simulink model "sysgenImageDoubleBuffer"  (Simulink 7.7)
settings: Solver=VariableStepDiscrete  StartTime=0.0  StopTime=((c_rx_rows_2*c_rx_cols_2)*2+(320*10))+5000  RelTol=1e-3
PreLoadFcn:
  | sysgenImageDoubleBuffer_PreLoadFcn
StartFcn:
  | tic;
undefined symbols (not defined in the file or in its folder): c_rx_cols_1, c_rx_cols_2, c_rx_rows_1, c_rx_rows_2, dpost_1, dpost_2
libraries: xbsIndex_r4 x160, dspbuff3 x6, dspsigattribs x6, dspmtrx3 x6, vipsrcs x2, simulink x2, xbsCopyrightNotice_r4 x1
(part 2 of 3)

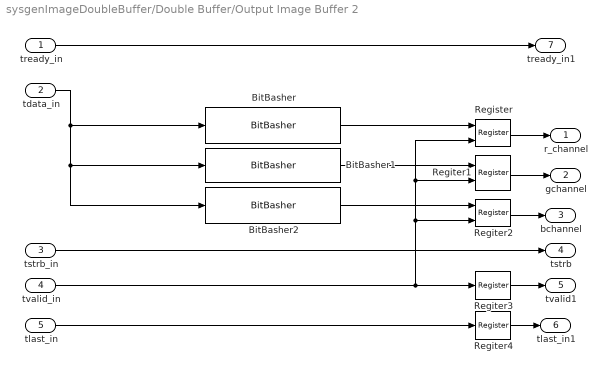
== system sysgenImageDoubleBuffer/Double Buffer/Output Image Buffer 2 ==
  tready_in : Inport
  tdata_in : Inport  Port=2
  tstrb_in : Inport  Port=3
  tvalid_in : Inport  Port=4
  tlast_in : Inport  Port=5
  BitBasher : xbsIndex_r4/BitBasher  bitexpr=|  display_expr=off  sr_1=1  arith_type1=Unsigned  bin_pt1=0  sr_2=2  arith_type2=Unsigned  bin_pt2=0  sr_3=3  arith_type3=Unsigned  bin_pt3=0  sr_4=4  arith_type4=Unsigned  bin_pt4=0  dbl_ovrd=off  block_type=bitbasher
      | <!DOCTYPE HTML PUBLIC "-//W3C//DTD HTML 4.0//EN" "http://www.w3.org/TR/REC-html40/strict.dtd">
      | <html><head><meta name="qrichtext" content="1" /><style type="text/css">
      | p, li { white-space: pre-wrap; }
      | </style></head><body style=" font-family:'MS Shell Dlg 2'; font-size:7.8pt; font-weight:400; font-style:normal;">
      | <p style=" margin-top:12px; margin-bottom:12px; margin-left:0px; margin-right:0px; -qt-block-indent:0; text-indent:0px;"><span style=" font-family:'MS Shell Dlg'; font-size:8pt;">r_channel={mem[23:16]}</span></p></body></html>
      settings: block_version=12.3
  BitBasher1 : xbsIndex_r4/BitBasher  bitexpr=|  display_expr=off  sr_1=1  arith_type1=Unsigned  bin_pt1=0  sr_2=2  arith_type2=Unsigned  bin_pt2=0  sr_3=3  arith_type3=Unsigned  bin_pt3=0  sr_4=4  arith_type4=Unsigned  bin_pt4=0  dbl_ovrd=off  block_type=bitbasher
      | <!DOCTYPE HTML PUBLIC "-//W3C//DTD HTML 4.0//EN" "http://www.w3.org/TR/REC-html40/strict.dtd">
      | <html><head><meta name="qrichtext" content="1" /><style type="text/css">
      | p, li { white-space: pre-wrap; }
      | </style></head><body style=" font-family:'MS Shell Dlg 2'; font-size:7.8pt; font-weight:400; font-style:normal;">
      | <p style=" margin-top:12px; margin-bottom:12px; margin-left:0px; margin-right:0px; -qt-block-indent:0; text-indent:0px;"><span style=" font-family:'MS Shell Dlg'; font-size:8pt;">g_channel={mem[15:8]}</span></p></body></html>
      settings: block_version=12.3
  BitBasher2 : xbsIndex_r4/BitBasher  bitexpr=|  display_expr=off  sr_1=1  arith_type1=Unsigned  bin_pt1=0  sr_2=2  arith_type2=Unsigned  bin_pt2=0  sr_3=3  arith_type3=Unsigned  bin_pt3=0  sr_4=4  arith_type4=Unsigned  bin_pt4=0  dbl_ovrd=off  block_type=bitbasher
      | <!DOCTYPE HTML PUBLIC "-//W3C//DTD HTML 4.0//EN" "http://www.w3.org/TR/REC-html40/strict.dtd">
      | <html><head><meta name="qrichtext" content="1" /><style type="text/css">
      | p, li { white-space: pre-wrap; }
      | </style></head><body style=" font-family:'MS Shell Dlg 2'; font-size:7.8pt; font-weight:400; font-style:normal;">
      | <p style=" margin-top:12px; margin-bottom:12px; margin-left:0px; margin-right:0px; -qt-block-indent:0; text-indent:0px;"><span style=" font-family:'MS Shell Dlg'; font-size:8pt;">b_channel={mem[7:0]}</span></p></body></html>
      settings: block_version=12.3
  Register : xbsIndex_r4/Register  init=0  rst=off  en=on  dbl_ovrd=off  block_type=register
      settings: block_version=12.3
  Regiter1 : xbsIndex_r4/Register  init=0  rst=off  en=on  dbl_ovrd=off  block_type=register
      settings: block_version=12.3
  Regiter2 : xbsIndex_r4/Register  init=0  rst=off  en=on  dbl_ovrd=off  block_type=register
      settings: block_version=12.3
  Regiter3 : xbsIndex_r4/Register  init=0  rst=off  en=off  dbl_ovrd=off  block_type=register
      settings: block_version=12.3
  Regiter4 : xbsIndex_r4/Register  init=0  rst=off  en=off  dbl_ovrd=off  block_type=register
      settings: block_version=12.3
  r_channel : Outport
  gchannel : Outport  Port=2
  bchannel : Outport  Port=3
  tstrb : Outport  Port=4
  tvalid1 : Outport  Port=5
  tlast_in1 : Outport  Port=6
  tready_in1 : Outport  Port=7
  wires:
  tready_in/1 -> tready_in1/1
  tvalid_in/1 -> Regiter2/2, Regiter1/2, Register/2, Regiter3/1
  tdata_in/1 -> BitBasher/1, BitBasher1/1, BitBasher2/1
  BitBasher/1 -> Register/1
  BitBasher1/1 -> Regiter1/1
  BitBasher2/1 -> Regiter2/1
  Register/1 -> r_channel/1
  Regiter1/1 -> gchannel/1
  Regiter2/1 -> bchannel/1
  Regiter3/1 -> tvalid1/1
  tlast_in/1 -> Regiter4/1
  Regiter4/1 -> tlast_in1/1
  tstrb_in/1 -> tstrb/1

== system sysgenImageDoubleBuffer/Image_Source_1/Image_source_1 ==
  valid_push : Inport
  valid_pop : Inport  Port=2
  B_Queue : dspbuff3/Queue  depth=9999999  trigger=Non-zero sample  overflow=Dynamic reallocation  pes=Warning  eso=off  fso=off  nso=off  clr=off  clrOutport=off  adf=on
  G_Queue : dspbuff3/Queue  depth=9999999  trigger=Non-zero sample  overflow=Dynamic reallocation  pes=Warning  eso=off  fso=off  nso=off  clr=off  clrOutport=off  adf=on
  R_Queue : dspbuff3/Queue  depth=9999999  trigger=Non-zero sample  overflow=Dynamic reallocation  pes=Warning  eso=off  fso=off  nso=off  clr=off  clrOutport=off  adf=on
  Subsystem1 : Subsystem
  r_channel : Outport
  g_channel : Outport  Port=2
  b_channel : Outport  Port=3
  wires:
  Subsystem1/1(r_channel) -> R_Queue/1
  Subsystem1/2(g_channel) -> G_Queue/1
  Subsystem1/3(b_channel) -> B_Queue/1
  R_Queue/1 -> r_channel/1
  G_Queue/1 -> g_channel/1
  B_Queue/1 -> b_channel/1
  valid_push/1 -> R_Queue/2, G_Queue/2, B_Queue/2
  valid_pop/1 -> R_Queue/3, G_Queue/3, B_Queue/3

== system sysgenImageDoubleBuffer/Image_Source_1/Subsystem1 ==
  ready : Inport
  aresetn : Inport  Port=2
  Data Type Conversion : DataTypeConversion
  Logical Operator : Logic  IconShape=distinctive  AllPortsSameDT=off
  Logical Operator1 : Logic  Operator=NOT  AllPortsSameDT=off  OutDataTypeStr=boolean
  Logical Operator2 : Logic  IconShape=distinctive  AllPortsSameDT=off
  image frame valid : Subsystem
  valid_push : Outport
  valid_pop : Outport  Port=2
  transmit_image_1 : Outport  Port=3
  wires:
  ready/1 -> Logical Operator/1
  Logical Operator/1 -> Data Type Conversion/1
  Logical Operator2/1 -> Logical Operator/2, Logical Operator1/1
  Logical Operator1/1 -> transmit_image_1/1
  Data Type Conversion/1 -> valid_pop/1
  image frame valid/1(Out1) -> Logical Operator2/1, valid_push/1
  aresetn/1 -> Logical Operator2/2

== system sysgenImageDoubleBuffer/image_Source_2/Subsystem ==
  ready : Inport
  aresetn : Inport  Port=2
  Data Type Conversion : DataTypeConversion
  Logical Operator : Logic  IconShape=distinctive  AllPortsSameDT=off
  Logical Operator1 : Logic  Operator=NOT  AllPortsSameDT=off  OutDataTypeStr=boolean
  Logical Operator2 : Logic  IconShape=distinctive  AllPortsSameDT=off
  image frame valid : Subsystem
  valid_push : Outport
  valid_pop : Outport  Port=2
  transmit_image_2 : Outport  Port=3
  wires:
  ready/1 -> Logical Operator/1
  Logical Operator/1 -> Data Type Conversion/1
  Logical Operator2/1 -> Logical Operator/2, Logical Operator1/1
  Logical Operator1/1 -> transmit_image_2/1
  Data Type Conversion/1 -> valid_pop/1
  aresetn/1 -> Logical Operator2/2
  image frame valid/1(Out1) -> Logical Operator2/1, valid_push/1

== system sysgenImageDoubleBuffer/image_Source_2/image_source_2 ==
  valid_push : Inport
  valid_pop : Inport  Port=2
  B_Queue : dspbuff3/Queue  depth=9999999  trigger=Non-zero sample  overflow=Dynamic reallocation  pes=Warning  eso=off  fso=off  nso=off  clr=off  clrOutport=off  adf=on
  G_Queue : dspbuff3/Queue  depth=9999999  trigger=Non-zero sample  overflow=Dynamic reallocation  pes=Warning  eso=off  fso=off  nso=off  clr=off  clrOutport=off  adf=on
  R_Queue : dspbuff3/Queue  depth=9999999  trigger=Non-zero sample  overflow=Dynamic reallocation  pes=Warning  eso=off  fso=off  nso=off  clr=off  clrOutport=off  adf=on
  Subsystem3 : Subsystem
  r_channel : Outport
  g_channel : Outport  Port=2
  b_channel : Outport  Port=3
  wires:
  Subsystem3/1(r_channel) -> R_Queue/1
  Subsystem3/2(g_channel) -> G_Queue/1
  Subsystem3/3(b_channel) -> B_Queue/1
  R_Queue/1 -> r_channel/1
  valid_push/1 -> R_Queue/2, G_Queue/2, B_Queue/2
  valid_pop/1 -> R_Queue/3, G_Queue/3, B_Queue/3
  G_Queue/1 -> g_channel/1
  B_Queue/1 -> b_channel/1

== system sysgenImageDoubleBuffer/Double Buffer/Double Buffer/Block Descriptor Generator ==
  note: This subsystem is composed of two units :
      | xldScatterGatherEngineLineTransfer : This unit interfaces with the Master AXI Read Channel
      | hence it provides a Slave AXI Read Channel. It provides data transfer commands in the form
      | of Block Descriptors to enable line transfers of the input image.
      | xldScatterGatherEngineBlockTransfer : This unit interfaces with the Master AXI Read Channel
      | hence it provides a Slave AXI Read Channel. It provides data transfer commands in the form
      | of Block Descriptors to enable Tile transfers of the input image.
  axi_read_channel_in : Inport
  image1_switch_to_transmit : Inport  Port=2
  Bus Creator3 : BusCreator  Inputs=5
  Constant : xbsIndex_r4/Constant  const=tx_rows_1  gui_display_data_type=Fixed-point  arith_type=Unsigned  n_bits=16  bin_pt=0  preci_type=Single  exp_width=8  frac_width=24  explicit_period=off  period=1  equ=P=C  opselect=C  inp2=PCIN>>17  opr=+  inp1=P  carry=CIN  dbl_ovrd=off  block_type=constant
      settings: block_version=12.3
  Constant2 : xbsIndex_r4/Constant  const=tx_cols_1  gui_display_data_type=Fixed-point  arith_type=Unsigned  n_bits=16  bin_pt=0  preci_type=Single  exp_width=8  frac_width=24  explicit_period=off  period=1  equ=P=C  opselect=C  inp2=PCIN>>17  opr=+  inp1=P  carry=CIN  dbl_ovrd=off  block_type=constant
      settings: block_version=12.3
  Demux2 : Demux  Outputs=8  BusSelectionMode=on
  Expression1 : xbsIndex_r4/Expression  expression=~a  align_bp=on  en=off  latency=0  precision=Full  arith_type=Unsigned  n_bits=16  bin_pt=0  dbl_ovrd=off  block_type=expr
      settings: block_version=13.4
  Receiver Block Descriptor Generator : xbsIndex_r4/MCode  mfname=xldScatterGatherEngineLineTransfer_1  explicit_period=on  period=1  inputsTable={'boundInpExpr'=>['','','','','','','','','rx_rows_1','rx_cols_1'],'inputs'=>['araddr','arlen','arsize','arburst','arprot','arcache','arvalid','rready','rx_rows','rx_cols']}  outputsTable={'outputs'=>['arready','rvalid','rlast','rdata','rresp'],'suppressOut'=>['off','off','off','off','off']}  dbl_ovrd=off  enable_stdout=off  enable_debug=off  suppress_output=on  defparams={'rx_rows',rx_rows_1,'rx_cols',rx_cols_1}  hide_port_list={}  block_type=mcode
      settings: block_version=12.3
  Subsystem : Subsystem
  Subsystem1 : Subsystem
  Subsystem4 : Subsystem
  Transmitter Block Descriptor Generator1 : xbsIndex_r4/MCode  mfname=xldScatterGatherEngineBlockTransfer_1  explicit_period=on  period=1  inputsTable={'boundInpExpr'=>['','','','','','','','','tx_rows_1','tx_cols_1'],'inputs'=>['araddr','arlen','arsize','arburst','arprot','arcache','arvalid','rready','tx_rows','tx_cols']}  outputsTable={'outputs'=>['arready','rvalid','rlast','rdata','rresp'],'suppressOut'=>['off','off','off','off','off']}  dbl_ovrd=off  enable_stdout=off  enable_debug=off  suppress_output=on  defparams={'tx_rows',tx_rows_1,'tx_cols',tx_cols_1}  hide_port_list={}  block_type=mcode
      settings: block_version=12.3
  axi_read_channel_out : Outport
  tx_rows_1 : Outport  Port=2
  tx_cols_1 : Outport  Port=3
  wires:
  image1_switch_to_transmit/1 -> Subsystem/1(gate), Subsystem1/1(gate), Expression1/1
  Subsystem/1(araddr) -> Receiver Block Descriptor Generator/1
  Subsystem/2(arlen) -> Receiver Block Descriptor Generator/2
  Subsystem/3(arsize) -> Receiver Block Descriptor Generator/3
  Subsystem/4(arburst) -> Receiver Block Descriptor Generator/4
  Subsystem/5(arprot) -> Receiver Block Descriptor Generator/5
  Subsystem/6(arcache) -> Receiver Block Descriptor Generator/6
  Subsystem/7(arvalid) -> Receiver Block Descriptor Generator/7
  Subsystem/8(rready) -> Receiver Block Descriptor Generator/8
  Demux2/1 -> Subsystem/2(araddr_in), Subsystem4/2(araddr_in)
  Demux2/2 -> Subsystem/3(arlen_in), Subsystem4/3(arlen_in)
  Demux2/3 -> Subsystem/4(arsize_in), Subsystem4/4(arsize_in)
  Demux2/4 -> Subsystem/5(arburst_in), Subsystem4/5(arburst_in)
  Demux2/5 -> Subsystem/6(arprot_in), Subsystem4/6(arprot_in)
  Demux2/6 -> Subsystem/7(arcache_in), Subsystem4/7(arcache_in)
  Demux2/7 -> Subsystem/8(arvalid_in), Subsystem4/8(arvalid_in)
  Demux2/8 -> Subsystem/9(rready_in), Subsystem4/9(rready_in)
  Subsystem4/1(araddr) -> Transmitter Block Descriptor Generator1/1
  Subsystem4/2(arlen) -> Transmitter Block Descriptor Generator1/2
  Subsystem4/3(arsize) -> Transmitter Block Descriptor Generator1/3
  Subsystem4/4(arburst) -> Transmitter Block Descriptor Generator1/4
  Subsystem4/5(arprot) -> Transmitter Block Descriptor Generator1/5
  Subsystem4/6(arcache) -> Transmitter Block Descriptor Generator1/6
  Subsystem4/7(arvalid) -> Transmitter Block Descriptor Generator1/7
  Subsystem4/8(rready) -> Transmitter Block Descriptor Generator1/8
  Receiver Block Descriptor Generator/1 -> Subsystem1/2(arready_1)
  Transmitter Block Descriptor Generator1/1 -> Subsystem1/7(arready_2)
  Receiver Block Descriptor Generator/2 -> Subsystem1/3(rvalid_1)
  Transmitter Block Descriptor Generator1/2 -> Subsystem1/8(rvalid_2)
  Receiver Block Descriptor Generator/3 -> Subsystem1/4(rlast_1)
  Transmitter Block Descriptor Generator1/3 -> Subsystem1/9(rlast_2)
  Receiver Block Descriptor Generator/4 -> Subsystem1/5(rdata_1)
  Transmitter Block Descriptor Generator1/4 -> Subsystem1/10(rdata_2)
  Transmitter Block Descriptor Generator1/5 -> Subsystem1/11(rresp_2)
  Receiver Block Descriptor Generator/5 -> Subsystem1/6(rresp_1)
  Subsystem1/1(arready) -> Bus Creator3/1
  Subsystem1/2(rvalid) -> Bus Creator3/2
  Subsystem1/3(rlast) -> Bus Creator3/3
  Subsystem1/4(rdata) -> Bus Creator3/4
  Subsystem1/5(rresp) -> Bus Creator3/5
  Bus Creator3/1 -> axi_read_channel_out/1
  axi_read_channel_in/1 -> Demux2/1
  Expression1/1 -> Subsystem4/1(gate)
  Constant/1 -> tx_rows_1/1
  Constant2/1 -> tx_cols_1/1

== system sysgenImageDoubleBuffer/Double Buffer/Double Buffer/Block Descriptor Generator1 ==
  note: This subsystem is composed of two units :
      | xldScatterGatherEngineLineTransfer : This unit interfaces with the Master AXI Read Channel
      | hence it provides a Slave AXI Read Channel. It provides data transfer commands in the form
      | of Block Descriptors to enable line transfers of the input image.
      | xldScatterGatherEngineBlockTransfer : This unit interfaces with the Master AXI Read Channel
      | hence it provides a Slave AXI Read Channel. It provides data transfer commands in the form
      | of Block Descriptors to enable Tile transfers of the input image.
  axi_read_channel_in : Inport
  image2_switch_to_transmit : Inport  Port=2
  Bus Creator3 : BusCreator  Inputs=5
  Constant3 : xbsIndex_r4/Constant  const=tx_rows_2  gui_display_data_type=Fixed-point  arith_type=Unsigned  n_bits=16  bin_pt=0  preci_type=Single  exp_width=8  frac_width=24  explicit_period=off  period=1  equ=P=C  opselect=C  inp2=PCIN>>17  opr=+  inp1=P  carry=CIN  dbl_ovrd=off  block_type=constant
      settings: block_version=12.3
  Constant4 : xbsIndex_r4/Constant  const=tx_cols_2  gui_display_data_type=Fixed-point  arith_type=Unsigned  n_bits=16  bin_pt=0  preci_type=Single  exp_width=8  frac_width=24  explicit_period=off  period=1  equ=P=C  opselect=C  inp2=PCIN>>17  opr=+  inp1=P  carry=CIN  dbl_ovrd=off  block_type=constant
      settings: block_version=12.3
  Constant7 : xbsIndex_r4/Constant  const=rx_rows_2  gui_display_data_type=Fixed-point  arith_type=Unsigned  n_bits=16  bin_pt=0  preci_type=Single  exp_width=8  frac_width=24  explicit_period=off  period=1  equ=P=C  opselect=C  inp2=PCIN>>17  opr=+  inp1=P  carry=CIN  dbl_ovrd=off  block_type=constant
      settings: block_version=12.3
  Constant8 : xbsIndex_r4/Constant  const=rx_cols_2  gui_display_data_type=Fixed-point  arith_type=Unsigned  n_bits=16  bin_pt=0  preci_type=Single  exp_width=8  frac_width=24  explicit_period=off  period=1  equ=P=C  opselect=C  inp2=PCIN>>17  opr=+  inp1=P  carry=CIN  dbl_ovrd=off  block_type=constant
      settings: block_version=12.3
  Demux2 : Demux  Outputs=8  BusSelectionMode=on
  Expression1 : xbsIndex_r4/Expression  expression=~a  align_bp=on  en=off  latency=0  precision=Full  arith_type=Unsigned  n_bits=16  bin_pt=0  dbl_ovrd=off  block_type=expr
      settings: block_version=13.4
  Receiver Block Descriptor Generator : xbsIndex_r4/MCode  mfname=xldScatterGatherEngineLineTransfer_2  explicit_period=on  period=1  inputsTable={'boundInpExpr'=>['','','','','','','','','rx_rows_2','rx_cols_2'],'inputs'=>['araddr','arlen','arsize','arburst','arprot','arcache','arvalid','rready','rx_rows','rx_cols']}  outputsTable={'outputs'=>['arready','rvalid','rlast','rdata','rresp'],'suppressOut'=>['off','off','off','off','off']}  dbl_ovrd=off  enable_stdout=off  enable_debug=off  suppress_output=on  defparams={'rx_rows',rx_rows_2,'rx_cols',rx_cols_2}  hide_port_list={}  block_type=mcode
      settings: block_version=12.3
  Subsystem : Subsystem
  Subsystem1 : Subsystem
  Subsystem4 : Subsystem
  Transmitter Block Descriptor Generator1 : xbsIndex_r4/MCode  mfname=xldScatterGatherEngineBlockTransfer_2  explicit_period=on  period=1  inputsTable={'boundInpExpr'=>['','','','','','','','','tx_rows_2','tx_cols_2','rx_rows_2','rx_cols_2'],'inputs'=>['araddr','arlen','arsize','arburst','arprot','arcache','arvalid','rready','tx_rows','tx_cols','rx_rows','rx_cols']}  outputsTable={'outputs'=>['arready','rvalid','rlast','rdata','rresp'],'suppressOut'=>['off','off','off','off','off']}  dbl_ovrd=off  enable_stdout=off  enable_debug=off  suppress_output=on  defparams={'tx_rows',tx_rows_2,'tx_cols',tx_cols_2,'rx_rows',rx_rows_2,'rx_cols',rx_cols_2}  hide_port_list={}  block_type=mcode
      settings: block_version=12.3
  axi_read_channel_out : Outport
  tx_rows_2 : Outport  Port=2
  tx_cols_2 : Outport  Port=3
  rx_rows_2 : Outport  Port=4
  rx_cols_2 : Outport  Port=5
  wires:
  image2_switch_to_transmit/1 -> Subsystem1/1(gate), Subsystem/1(gate), Expression1/1
  Subsystem/1(araddr) -> Receiver Block Descriptor Generator/1
  Subsystem/2(arlen) -> Receiver Block Descriptor Generator/2
  Subsystem/3(arsize) -> Receiver Block Descriptor Generator/3
  Subsystem/4(arburst) -> Receiver Block Descriptor Generator/4
  Subsystem/5(arprot) -> Receiver Block Descriptor Generator/5
  Subsystem/6(arcache) -> Receiver Block Descriptor Generator/6
  Subsystem/7(arvalid) -> Receiver Block Descriptor Generator/7
  Subsystem/8(rready) -> Receiver Block Descriptor Generator/8
  Demux2/1 -> Subsystem/2(araddr_in), Subsystem4/2(araddr_in)
  Demux2/2 -> Subsystem/3(arlen_in), Subsystem4/3(arlen_in)
  Demux2/3 -> Subsystem/4(arsize_in), Subsystem4/4(arsize_in)
  Demux2/4 -> Subsystem/5(arburst_in), Subsystem4/5(arburst_in)
  Demux2/5 -> Subsystem/6(arprot_in), Subsystem4/6(arprot_in)
  Demux2/6 -> Subsystem/7(arcache_in), Subsystem4/7(arcache_in)
  Demux2/7 -> Subsystem/8(arvalid_in), Subsystem4/8(arvalid_in)
  Demux2/8 -> Subsystem/9(rready_in), Subsystem4/9(rready_in)
  Subsystem4/1(araddr) -> Transmitter Block Descriptor Generator1/1
  Subsystem4/2(arlen) -> Transmitter Block Descriptor Generator1/2
  Subsystem4/3(arsize) -> Transmitter Block Descriptor Generator1/3
  Subsystem4/4(arburst) -> Transmitter Block Descriptor Generator1/4
  Subsystem4/5(arprot) -> Transmitter Block Descriptor Generator1/5
  Subsystem4/6(arcache) -> Transmitter Block Descriptor Generator1/6
  Subsystem4/7(arvalid) -> Transmitter Block Descriptor Generator1/7
  Subsystem4/8(rready) -> Transmitter Block Descriptor Generator1/8
  Receiver Block Descriptor Generator/1 -> Subsystem1/2(arready_1)
  Transmitter Block Descriptor Generator1/1 -> Subsystem1/7(arready_2)
  Receiver Block Descriptor Generator/2 -> Subsystem1/3(rvalid_1)
  Transmitter Block Descriptor Generator1/2 -> Subsystem1/8(rvalid_2)
  Receiver Block Descriptor Generator/3 -> Subsystem1/4(rlast_1)
  Transmitter Block Descriptor Generator1/3 -> Subsystem1/9(rlast_2)
  Receiver Block Descriptor Generator/4 -> Subsystem1/5(rdata_1)
  Transmitter Block Descriptor Generator1/4 -> Subsystem1/10(rdata_2)
  Transmitter Block Descriptor Generator1/5 -> Subsystem1/11(rresp_2)
  Receiver Block Descriptor Generator/5 -> Subsystem1/6(rresp_1)
  Subsystem1/1(arready) -> Bus Creator3/1
  Subsystem1/2(rvalid) -> Bus Creator3/2
  Subsystem1/3(rlast) -> Bus Creator3/3
  Subsystem1/4(rdata) -> Bus Creator3/4
  Subsystem1/5(rresp) -> Bus Creator3/5
  Bus Creator3/1 -> axi_read_channel_out/1
  axi_read_channel_in/1 -> Demux2/1
  Expression1/1 -> Subsystem4/1(gate)
  Constant3/1 -> tx_rows_2/1
  Constant4/1 -> tx_cols_2/1
  Constant7/1 -> rx_rows_2/1
  Constant8/1 -> rx_cols_2/1

== system sysgenImageDoubleBuffer/Double Buffer/Double Buffer/Control Instructions Generator ==
  note: This block configures the VDMA as Reciever and
      | then as transmitter of image data. It interfaces with
      |  the Slave AXI Lite control interface of the VDMA,
      | hence it provides an Master AXI Lite Interface
  axi_lite_channel_in : Inport
  image1_switch_to_transmit : Inport  Port=2
  aresetn : Inport  Port=3
  Bus Creator1 : BusCreator  Inputs=8
  Control Command Generator : xbsIndex_r4/MCode  mfname=xlWriteControlRegister_db  explicit_period=on  period=1  inputsTable={'boundInpExpr'=>['','','','','','','','','',''],'inputs'=>['awready','wready','bresp','bvalid','arready','rvalid','rdata','rresp','switch_to_transmit','aresetn']}  outputsTable={'outputs'=>['awvalid','awaddr','wvalid','wdata','bready','arvalid','araddr','rready'],'suppressOut'=>['off','off','off','off','off','off','off','off']}  dbl_ovrd=off  enable_stdout=off  enable_debug=off  suppress_output=on  defparams={}  hide_port_list={}  block_type=mcode
      settings: block_version=12.3
  Demux : Demux  Outputs=8  BusSelectionMode=on
  axi_lite_channel_out : Outport
  wires:
  Demux/1 -> Control Command Generator/1
  Demux/2 -> Control Command Generator/2
  Demux/3 -> Control Command Generator/3
  Demux/4 -> Control Command Generator/4
  Demux/5 -> Control Command Generator/5
  Demux/6 -> Control Command Generator/6
  Demux/7 -> Control Command Generator/7
  Demux/8 -> Control Command Generator/8
  Control Command Generator/1 -> Bus Creator1/1
  Control Command Generator/2 -> Bus Creator1/2
  Control Command Generator/3 -> Bus Creator1/3
  Control Command Generator/4 -> Bus Creator1/4
  Control Command Generator/5 -> Bus Creator1/5
  Control Command Generator/6 -> Bus Creator1/6
  Control Command Generator/7 -> Bus Creator1/7
  Control Command Generator/8 -> Bus Creator1/8
  image1_switch_to_transmit/1 -> Control Command Generator/9
  axi_lite_channel_in/1 -> Demux/1
  Bus Creator1/1 -> axi_lite_channel_out/1
  aresetn/1 -> Control Command Generator/10

== system sysgenImageDoubleBuffer/Double Buffer/Double Buffer/Control Instructions Generator1 ==
  note: This block configures the VDMA as Reciever and
      | then as transmitter of image data. It interfaces with
      |  the Slave AXI Lite control interface of the VDMA,
      | hence it provides an Master AXI Lite Interface
  axi_lite_channel_in : Inport
  image2_switch_to_transmit : Inport  Port=2
  aresetn : Inport  Port=3
  Bus Creator1 : BusCreator  Inputs=8
  Control Command Generator : xbsIndex_r4/MCode  mfname=xlWriteControlRegister_db  explicit_period=on  period=1  inputsTable={'boundInpExpr'=>['','','','','','','','','',''],'inputs'=>['awready','wready','bresp','bvalid','arready','rvalid','rdata','rresp','switch_to_transmit','aresetn']}  outputsTable={'outputs'=>['awvalid','awaddr','wvalid','wdata','bready','arvalid','araddr','rready'],'suppressOut'=>['off','off','off','off','off','off','off','off']}  dbl_ovrd=off  enable_stdout=off  enable_debug=off  suppress_output=on  defparams={}  hide_port_list={}  block_type=mcode
      settings: block_version=12.3
  Demux : Demux  Outputs=8  BusSelectionMode=on
  axi_lite_channel_out : Outport
  wires:
  Demux/1 -> Control Command Generator/1
  Demux/2 -> Control Command Generator/2
  Demux/3 -> Control Command Generator/3
  Demux/4 -> Control Command Generator/4
  Demux/5 -> Control Command Generator/5
  Demux/6 -> Control Command Generator/6
  Demux/7 -> Control Command Generator/7
  Demux/8 -> Control Command Generator/8
  Control Command Generator/1 -> Bus Creator1/1
  Control Command Generator/2 -> Bus Creator1/2
  Control Command Generator/3 -> Bus Creator1/3
  Control Command Generator/4 -> Bus Creator1/4
  Control Command Generator/5 -> Bus Creator1/5
  Control Command Generator/6 -> Bus Creator1/6
  Control Command Generator/7 -> Bus Creator1/7
  Control Command Generator/8 -> Bus Creator1/8
  axi_lite_channel_in/1 -> Demux/1
  Bus Creator1/1 -> axi_lite_channel_out/1
  aresetn/1 -> Control Command Generator/10
  image2_switch_to_transmit/1 -> Control Command Generator/9

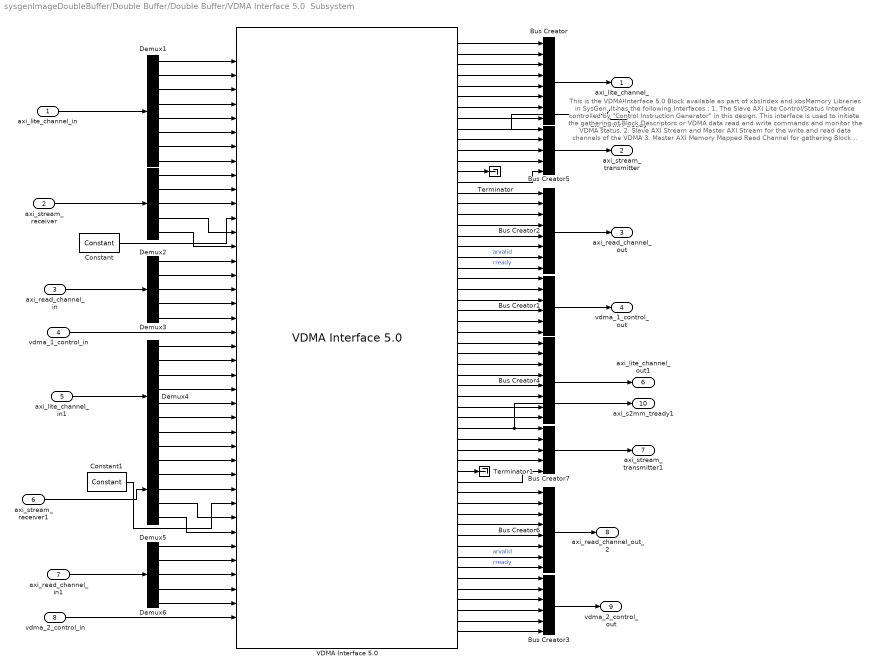
== system sysgenImageDoubleBuffer/Double Buffer/Double Buffer/VDMA Interface 5.0  Subsystem ==
  note: This is the VDMA Interface 5.0  Block available as part of xbsIndex and xbsMemory Libraries
      | in SysGen. It has the following Interfaces :
      |
      |    1. The Slave AXI Lite Control/Status Interface controlled by "Control Instruction Generator"
      |        in this design. This interface is used to initiate the gathering of Block Descriptors or VDMA
      |        data read and write commands and monitor the VDMA status.
      |
      |     2. Slave AXI Stream and Master AXI Stream for the write and read data channels of the VDMA
      |
      |     3. Master AXI Memory Mapped Read Channel for gathering Block Descriptor for the VDMA.
      |         In this design the block descriptors are provided by Block Descriptor Generator.
      |
      | On netlisting this block is transformed into top level Gateway Ins and Gateway Outs hence the
      | color of the block is yellow.
  axi_lite_channel_in : Inport
  axi_stream_receiver : Inport  Port=2
  axi_read_channel_in : Inport  Port=3
  vdma_1_control_in : Inport  Port=4
  axi_lite_channel_in1 : Inport  Port=5
  axi_stream_receiver1 : Inport  Port=6
  axi_read_channel_in1 : Inport  Port=7
  vdma_2_control_in : Inport  Port=8
  Bus Creator{,2,4,6} (4 alike) : BusCreator  Inputs=8
  Bus Creator1 : BusCreator  Inputs=6
  Bus Creator3 : BusCreator  Inputs=6
  Bus Creator5 : BusCreator  Inputs=5
  Bus Creator7 : BusCreator  Inputs=5
  Constant : xbsIndex_r4/Constant  const=0  gui_display_data_type=Fixed-point  arith_type=Unsigned  n_bits=1  bin_pt=0  preci_type=Single  exp_width=8  frac_width=24  explicit_period=on  period=1  equ=P=C  opselect=C  inp2=PCIN>>17  opr=+  inp1=P  carry=CIN  dbl_ovrd=off  block_type=constant
  Constant1 : xbsIndex_r4/Constant  const=0  gui_display_data_type=Fixed-point  arith_type=Unsigned  n_bits=1  bin_pt=0  preci_type=Single  exp_width=8  frac_width=24  explicit_period=on  period=1  equ=P=C  opselect=C  inp2=PCIN>>17  opr=+  inp1=P  carry=CIN  dbl_ovrd=off  block_type=constant
  Demux1 : Demux  Outputs=8  BusSelectionMode=on
  Demux{2..3,5..6} (4 alike) : Demux  Outputs=5  BusSelectionMode=on
  Demux4 : Demux  Outputs=8  BusSelectionMode=on
  Terminator : Terminator
  Terminator1 : Terminator
  "VDMA Interface 5.0 " : xbsIndex_r4/VDMA Interface 5.0   c_mem_size=64MB  c_number_of_vdma_if=2  c_stream_if_configuration_1=Master/Slave  c_no_of_frames_1=1  c_use_fsync_1=off  c_flush_on_fsync_1=off  c_use_sg_engine_1=on  c_video_prm_read_1=on  c_m_axis_mm2s_data_width_1=32  c_m_axis_mm2s_frame_sync_tuser_1=off  c_mm2s_linebuffer_depth_1=0  c_mm2s_linebuffer_threshold_1=1  c_s_axis_s2mm_data_width_1=32  c_s_axis_s2mm_frame_sync_tuser_1=off  c_s2mm_linebuffer_depth_1=0  c_s2mm_linebuffer_threshold_1=1  c_stream_if_configuration_2=Master/Slave  c_no_of_frames_2=1  c_use_fsync_2=off  c_flush_on_fsync_2=off  c_use_sg_engine_2=on  c_video_prm_read_2=on  c_m_axis_mm2s_data_width_2=32  c_m_axis_mm2s_frame_sync_tuser_2=off  c_mm2s_linebuffer_depth_2=0  c_mm2s_linebuffer_threshold_2=1  c_s_axis_s2mm_data_width_2=32  c_s_axis_s2mm_frame_sync_tuser_2=off  c_s2mm_linebuffer_depth_2=0  c_s2mm_linebuffer_threshold_2=1  c_stream_if_configuration_3=Master/Slave  c_no_of_frames_3=3  c_use_fsync_3=off  c_flush_on_fsync_3=off  c_use_sg_engine_3=off  c_video_prm_read_3=on  c_m_axis_mm2s_data_width_3=32  c_m_axis_mm2s_frame_sync_tuser_3=off  c_mm2s_linebuffer_depth_3=0  c_mm2s_linebuffer_threshold_3=1  c_s_axis_s2mm_data_width_3=32  c_s_axis_s2mm_frame_sync_tuser_3=off  c_s2mm_linebuffer_depth_3=0  c_s2mm_linebuffer_threshold_3=1  c_stream_if_configuration_4=Master/Slave  c_no_of_frames_4=3  c_use_fsync_4=off  c_flush_on_fsync_4=off  c_use_sg_engine_4=off  c_video_prm_read_4=on  c_m_axis_mm2s_data_width_4=32  c_m_axis_mm2s_frame_sync_tuser_4=off  c_mm2s_linebuffer_depth_4=0  c_mm2s_linebuffer_threshold_4=1  c_s_axis_s2mm_data_width_4=32  c_s_axis_s2mm_frame_sync_tuser_4=off  c_s2mm_linebuffer_depth_4=0  c_s2mm_linebuffer_threshold_4=1  simulation_model='emi_v5_0:EMI_v5_0_Model'  block_type=vdma
      settings: infoedit="This is a bit-accurate simulation model for multiple AXI VDMA external memory interfaces.  Netlisting will generate the port interface that can be attached to the VDMA IP.  This block is currently in beta."
  axi_lite_channel_out : Outport
  axi_stream_transmitter : Outport  Port=2
  axi_read_channel_out : Outport  Port=3
  vdma_1_control_out : Outport  Port=4
  axi_s2mm_tready : Outport  Port=5
  axi_lite_channel_out1 : Outport  Port=6
  axi_stream_transmitter1 : Outport  Port=7
  axi_read_channel_out_2 : Outport  Port=8
  vdma_2_control_out : Outport  Port=9
  axi_s2mm_tready1 : Outport  Port=10
  wires:
  axi_read_channel_in/1 -> Demux3/1
  axi_lite_channel_in/1 -> Demux1/1
  Bus Creator5/1 -> axi_stream_transmitter/1
  axi_stream_receiver/1 -> Demux2/1
  Bus Creator2/1 -> axi_read_channel_out/1
  "VDMA Interface 5.0 "/1 -> Bus Creator/1
  "VDMA Interface 5.0 "/2 -> Bus Creator/2
  "VDMA Interface 5.0 "/3 -> Bus Creator/3
  "VDMA Interface 5.0 "/4 -> Bus Creator/4
  "VDMA Interface 5.0 "/5 -> Bus Creator/5
  "VDMA Interface 5.0 "/6 -> Bus Creator/6
  "VDMA Interface 5.0 "/7 -> Bus Creator/7
  "VDMA Interface 5.0 "/8 -> Bus Creator/8
  "VDMA Interface 5.0 "/9 -> Bus Creator5/1, axi_s2mm_tready/1
  "VDMA Interface 5.0 "/10 -> Bus Creator5/2
  "VDMA Interface 5.0 "/11 -> Bus Creator5/3
  "VDMA Interface 5.0 "/12 -> Bus Creator5/4
  "VDMA Interface 5.0 "/14 -> Bus Creator5/5
  "VDMA Interface 5.0 "/15 -> Bus Creator2/1
  "VDMA Interface 5.0 "/16 -> Bus Creator2/2
  "VDMA Interface 5.0 "/17 -> Bus Creator2/3
  "VDMA Interface 5.0 "/18 -> Bus Creator2/4
  "VDMA Interface 5.0 "/19 -> Bus Creator2/5
  "VDMA Interface 5.0 "/20 -> Bus Creator2/6
  "VDMA Interface 5.0 "/21 -> Bus Creator2/7  "arvalid"
  "VDMA Interface 5.0 "/22 -> Bus Creator2/8  "rready"
  "VDMA Interface 5.0 "/23 -> Bus Creator1/1
  "VDMA Interface 5.0 "/24 -> Bus Creator1/2
  "VDMA Interface 5.0 "/25 -> Bus Creator1/3
  "VDMA Interface 5.0 "/26 -> Bus Creator1/4
  "VDMA Interface 5.0 "/27 -> Bus Creator1/5
  "VDMA Interface 5.0 "/28 -> Bus Creator1/6
  "VDMA Interface 5.0 "/51 -> Bus Creator3/1
  "VDMA Interface 5.0 "/52 -> Bus Creator3/2
  "VDMA Interface 5.0 "/53 -> Bus Creator3/3
  "VDMA Interface 5.0 "/54 -> Bus Creator3/4
  "VDMA Interface 5.0 "/55 -> Bus Creator3/5
  "VDMA Interface 5.0 "/56 -> Bus Creator3/6
  "VDMA Interface 5.0 "/29 -> Bus Creator4/1
  "VDMA Interface 5.0 "/30 -> Bus Creator4/2
  "VDMA Interface 5.0 "/31 -> Bus Creator4/3
  "VDMA Interface 5.0 "/32 -> Bus Creator4/4
  "VDMA Interface 5.0 "/33 -> Bus Creator4/5
  "VDMA Interface 5.0 "/34 -> Bus Creator4/6
  "VDMA Interface 5.0 "/35 -> Bus Creator4/7
  "VDMA Interface 5.0 "/36 -> Bus Creator4/8
  "VDMA Interface 5.0 "/37 -> axi_s2mm_tready1/1, Bus Creator7/1
  "VDMA Interface 5.0 "/38 -> Bus Creator7/2
  "VDMA Interface 5.0 "/39 -> Bus Creator7/3
  "VDMA Interface 5.0 "/42 -> Bus Creator7/5
  "VDMA Interface 5.0 "/43 -> Bus Creator6/1
  "VDMA Interface 5.0 "/44 -> Bus Creator6/2
  "VDMA Interface 5.0 "/45 -> Bus Creator6/3
  "VDMA Interface 5.0 "/46 -> Bus Creator6/4
  "VDMA Interface 5.0 "/47 -> Bus Creator6/5
  "VDMA Interface 5.0 "/48 -> Bus Creator6/6
  "VDMA Interface 5.0 "/49 -> Bus Creator6/7  "arvalid"
  "VDMA Interface 5.0 "/50 -> Bus Creator6/8  "rready"
  Bus Creator6/1 -> axi_read_channel_out_2/1
  Bus Creator7/1 -> axi_stream_transmitter1/1
  Bus Creator4/1 -> axi_lite_channel_out1/1
  Bus Creator/1 -> axi_lite_channel_out/1
  axi_lite_channel_in1/1 -> Demux4/1
  axi_read_channel_in1/1 -> Demux6/1
  axi_stream_receiver1/1 -> Demux5/1
  Bus Creator1/1 -> vdma_1_control_out/1
  Bus Creator3/1 -> vdma_2_control_out/1
  Demux1/1 -> "VDMA Interface 5.0 "/1
  Demux1/2 -> "VDMA Interface 5.0 "/2
  Demux1/3 -> "VDMA Interface 5.0 "/3
  Demux1/4 -> "VDMA Interface 5.0 "/4
  Demux1/5 -> "VDMA Interface 5.0 "/5
  Demux1/6 -> "VDMA Interface 5.0 "/6
  Demux1/7 -> "VDMA Interface 5.0 "/7
  Demux1/8 -> "VDMA Interface 5.0 "/8
  Demux2/1 -> "VDMA Interface 5.0 "/9
  Demux2/2 -> "VDMA Interface 5.0 "/10
  Demux2/3 -> "VDMA Interface 5.0 "/11
  Demux3/1 -> "VDMA Interface 5.0 "/15
  Demux3/2 -> "VDMA Interface 5.0 "/16
  Demux3/3 -> "VDMA Interface 5.0 "/17
  Demux3/4 -> "VDMA Interface 5.0 "/18
  Demux3/5 -> "VDMA Interface 5.0 "/19
  Demux4/1 -> "VDMA Interface 5.0 "/21
  Demux4/2 -> "VDMA Interface 5.0 "/22
  Demux4/3 -> "VDMA Interface 5.0 "/23
  Demux4/4 -> "VDMA Interface 5.0 "/24
  Demux4/5 -> "VDMA Interface 5.0 "/25
  Demux4/6 -> "VDMA Interface 5.0 "/26
  Demux4/7 -> "VDMA Interface 5.0 "/27
  Demux4/8 -> "VDMA Interface 5.0 "/28
  Demux6/1 -> "VDMA Interface 5.0 "/35
  Demux6/2 -> "VDMA Interface 5.0 "/36
  Demux6/3 -> "VDMA Interface 5.0 "/37
  Demux6/4 -> "VDMA Interface 5.0 "/38
  Demux6/5 -> "VDMA Interface 5.0 "/39
  vdma_1_control_in/1 -> "VDMA Interface 5.0 "/20
  vdma_2_control_in/1 -> "VDMA Interface 5.0 "/40
  Constant/1 -> "VDMA Interface 5.0 "/12
  Demux2/4 -> "VDMA Interface 5.0 "/13
  Demux2/5 -> "VDMA Interface 5.0 "/14
  Demux5/1 -> "VDMA Interface 5.0 "/29
  Demux5/2 -> "VDMA Interface 5.0 "/30
  Demux5/3 -> "VDMA Interface 5.0 "/31
  Demux5/4 -> "VDMA Interface 5.0 "/33
  Demux5/5 -> "VDMA Interface 5.0 "/34
  Constant1/1 -> "VDMA Interface 5.0 "/32
  "VDMA Interface 5.0 "/13 -> Terminator/1
  "VDMA Interface 5.0 "/41 -> Terminator1/1
  "VDMA Interface 5.0 "/40 -> Bus Creator7/4

== system sysgenImageDoubleBuffer/Image_Source_1/Image_source_1/Subsystem1 ==
  Data Type Conversion : DataTypeConversion  OutDataTypeStr=double
  Data Type Conversion1 : DataTypeConversion  OutDataTypeStr=double
  Data Type Conversion2 : DataTypeConversion  OutDataTypeStr=double
  Image From File : vipsrcs/Image From File  Tag=vipblks_nd  SystemSampleTime=-1  FileName=./lion.bmp  imagePorts=Separate color signals  Ts=c_rx_rows_1*c_rx_cols_1  ImageDataType=uint8  Signed=on  WordLength=16  sdImageDataType=uint(8)  FractionLengthMode=User-defined  FractionLength=15  OutPortLabels=R|G|B
  pixelize : Subsystem
  pixelize1 : Subsystem
  pixelize2 : Subsystem
  r_channel : Outport
  g_channel : Outport  Port=2
  b_channel : Outport  Port=3
  wires:
  Image From File/1 -> pixelize/1(In1)
  Image From File/2 -> pixelize1/1(In1)
  Image From File/3 -> pixelize2/1(In1)
  pixelize/1(Out1) -> Data Type Conversion/1
  pixelize1/1(Out1) -> Data Type Conversion1/1
  pixelize2/1(Out1) -> Data Type Conversion2/1
  Data Type Conversion/1 -> r_channel/1
  Data Type Conversion1/1 -> g_channel/1
  Data Type Conversion2/1 -> b_channel/1

== system sysgenImageDoubleBuffer/Image_Source_1/Subsystem1/image frame valid ==
  Constant2 : Constant  Value=0
  Constant3 : Constant
  Counter Free-Running : simulink/Sources/Counter Free-Running  SystemSampleTime=-1  NumBits=32  tsamp=-1
  Switch : Switch  Threshold=c_rx_rows_1*c_rx_cols_1+(c_rx_rows_1*30)
  Out1 : Outport
  wires:
  Constant2/1 -> Switch/1
  Counter Free-Running/1 -> Switch/2
  Constant3/1 -> Switch/3
  Switch/1 -> Out1/1

== system sysgenImageDoubleBuffer/image_Source_2/Subsystem/image frame valid ==
  Constant2 : Constant  Value=0
  Constant3 : Constant
  Counter Free-Running : simulink/Sources/Counter Free-Running  SystemSampleTime=-1  NumBits=32  tsamp=-1
  Switch : Switch  Threshold=(c_rx_rows_2*c_rx_cols_2)+(c_rx_rows_2*30)
  Out1 : Outport
  wires:
  Switch/1 -> Out1/1
  Constant3/1 -> Switch/3
  Counter Free-Running/1 -> Switch/2
  Constant2/1 -> Switch/1

== system sysgenImageDoubleBuffer/image_Source_2/image_source_2/Subsystem3 ==
  Data Type Conversion : DataTypeConversion  OutDataTypeStr=double
  Data Type Conversion1 : DataTypeConversion  OutDataTypeStr=double
  Data Type Conversion2 : DataTypeConversion  OutDataTypeStr=double
  Image From File : vipsrcs/Image From File  Tag=vipblks_nd  SystemSampleTime=-1  FileName=./leopard.bmp  imagePorts=Separate color signals  Ts=c_rx_rows_2*c_rx_cols_2  ImageDataType=uint8  Signed=on  WordLength=16  sdImageDataType=uint(8)  FractionLengthMode=User-defined  FractionLength=15  OutPortLabels=R|G|B
  pixelize : Subsystem
  pixelize1 : Subsystem
  pixelize2 : Subsystem
  r_channel : Outport
  g_channel : Outport  Port=2
  b_channel : Outport  Port=3
  wires:
  Image From File/1 -> pixelize/1(In1)
  Image From File/2 -> pixelize1/1(In1)
  Image From File/3 -> pixelize2/1(In1)
  pixelize/1(Out1) -> Data Type Conversion/1
  pixelize1/1(Out1) -> Data Type Conversion1/1
  pixelize2/1(Out1) -> Data Type Conversion2/1
  Data Type Conversion/1 -> r_channel/1
  Data Type Conversion1/1 -> g_channel/1
  Data Type Conversion2/1 -> b_channel/1

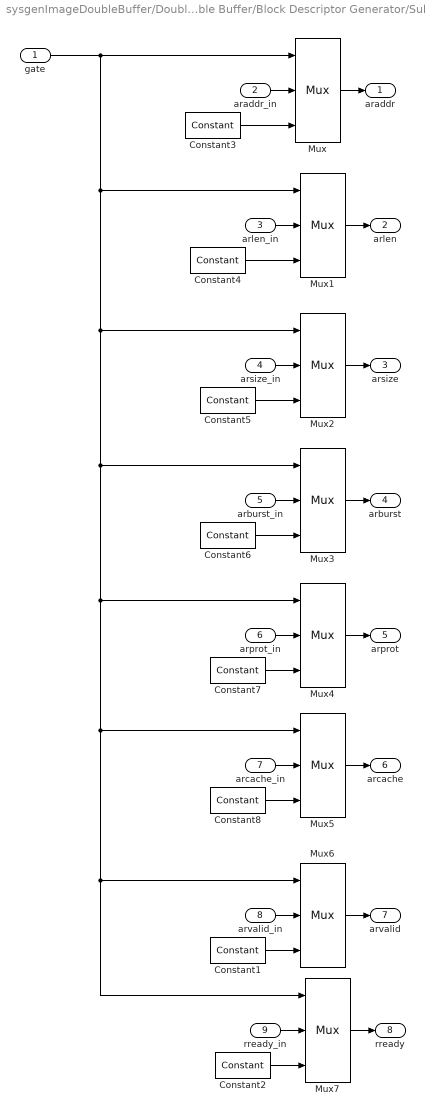
== system sysgenImageDoubleBuffer/Double Buffer/Double Buffer/Block Descriptor Generator/Subsystem ==
  gate : Inport
  araddr_in : Inport  Port=2
  arlen_in : Inport  Port=3
  arsize_in : Inport  Port=4
  arburst_in : Inport  Port=5
  arprot_in : Inport  Port=6
  arcache_in : Inport  Port=7
  arvalid_in : Inport  Port=8
  rready_in : Inport  Port=9
  Constant1 : xbsIndex_r4/Constant  const=0  gui_display_data_type=Fixed-point  arith_type=Boolean  n_bits=4  bin_pt=0  preci_type=Single  exp_width=8  frac_width=24  explicit_period=off  period=1  equ=P=C  opselect=C  inp2=PCIN>>17  opr=+  inp1=P  carry=CIN  dbl_ovrd=off  block_type=constant
      settings: block_version=12.3
  Constant2 : xbsIndex_r4/Constant  const=0  gui_display_data_type=Fixed-point  arith_type=Boolean  n_bits=4  bin_pt=0  preci_type=Single  exp_width=8  frac_width=24  explicit_period=off  period=1  equ=P=C  opselect=C  inp2=PCIN>>17  opr=+  inp1=P  carry=CIN  dbl_ovrd=off  block_type=constant
      settings: block_version=12.3
  Constant3 : xbsIndex_r4/Constant  const=0  gui_display_data_type=Fixed-point  arith_type=Unsigned  n_bits=32  bin_pt=0  preci_type=Single  exp_width=8  frac_width=24  explicit_period=off  period=1  equ=P=C  opselect=C  inp2=PCIN>>17  opr=+  inp1=P  carry=CIN  dbl_ovrd=off  block_type=constant
      settings: block_version=12.3
  Constant4 : xbsIndex_r4/Constant  const=0  gui_display_data_type=Fixed-point  arith_type=Unsigned  n_bits=8  bin_pt=0  preci_type=Single  exp_width=8  frac_width=24  explicit_period=off  period=1  equ=P=C  opselect=C  inp2=PCIN>>17  opr=+  inp1=P  carry=CIN  dbl_ovrd=off  block_type=constant
      settings: block_version=12.3
  Constant5 : xbsIndex_r4/Constant  const=0  gui_display_data_type=Fixed-point  arith_type=Unsigned  n_bits=3  bin_pt=0  preci_type=Single  exp_width=8  frac_width=24  explicit_period=off  period=1  equ=P=C  opselect=C  inp2=PCIN>>17  opr=+  inp1=P  carry=CIN  dbl_ovrd=off  block_type=constant
      settings: block_version=12.3
  Constant6 : xbsIndex_r4/Constant  const=0  gui_display_data_type=Fixed-point  arith_type=Unsigned  n_bits=2  bin_pt=0  preci_type=Single  exp_width=8  frac_width=24  explicit_period=off  period=1  equ=P=C  opselect=C  inp2=PCIN>>17  opr=+  inp1=P  carry=CIN  dbl_ovrd=off  block_type=constant
      settings: block_version=12.3
  Constant7 : xbsIndex_r4/Constant  const=0  gui_display_data_type=Fixed-point  arith_type=Unsigned  n_bits=3  bin_pt=0  preci_type=Single  exp_width=8  frac_width=24  explicit_period=off  period=1  equ=P=C  opselect=C  inp2=PCIN>>17  opr=+  inp1=P  carry=CIN  dbl_ovrd=off  block_type=constant
      settings: block_version=12.3
  Constant8 : xbsIndex_r4/Constant  const=0  gui_display_data_type=Fixed-point  arith_type=Unsigned  n_bits=4  bin_pt=0  preci_type=Single  exp_width=8  frac_width=24  explicit_period=off  period=1  equ=P=C  opselect=C  inp2=PCIN>>17  opr=+  inp1=P  carry=CIN  dbl_ovrd=off  block_type=constant
      settings: block_version=12.3
  Mux{,1..7} (8 alike) : xbsIndex_r4/Mux  inputs=2  en=off  latency=0  precision=Full  arith_type=Unsigned  n_bits=16  bin_pt=14  quantization=Truncate  overflow=Wrap  dbl_ovrd=off  block_type=mux
      settings: block_version=12.3
  araddr : Outport
  arlen : Outport  Port=2
  arsize : Outport  Port=3
  arburst : Outport  Port=4
  arprot : Outport  Port=5
  arcache : Outport  Port=6
  arvalid : Outport  Port=7
  rready : Outport  Port=8
  wires:
  Constant3/1 -> Mux/3
  Constant4/1 -> Mux1/3
  Constant5/1 -> Mux2/3
  Constant6/1 -> Mux3/3
  Constant7/1 -> Mux4/3
  Constant8/1 -> Mux5/3
  gate/1 -> Mux/1, Mux1/1, Mux2/1, Mux3/1, Mux4/1, Mux5/1, Mux6/1, Mux7/1
  araddr_in/1 -> Mux/2
  Mux/1 -> araddr/1
  arlen_in/1 -> Mux1/2
  Mux1/1 -> arlen/1
  arsize_in/1 -> Mux2/2
  Mux2/1 -> arsize/1
  arburst_in/1 -> Mux3/2
  Mux3/1 -> arburst/1
  arprot_in/1 -> Mux4/2
  Mux4/1 -> arprot/1
  arcache_in/1 -> Mux5/2
  Mux5/1 -> arcache/1
  Constant1/1 -> Mux6/3
  arvalid_in/1 -> Mux6/2
  Mux6/1 -> arvalid/1
  Constant2/1 -> Mux7/3
  rready_in/1 -> Mux7/2
  Mux7/1 -> rready/1

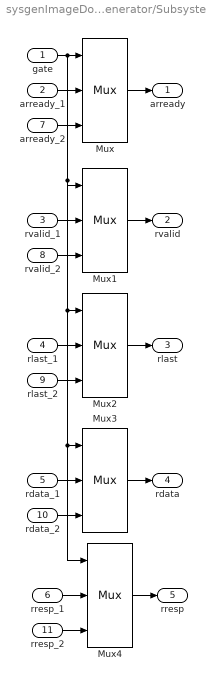
== system sysgenImageDoubleBuffer/Double Buffer/Double Buffer/Block Descriptor Generator/Subsystem1 ==
  gate : Inport
  arready_1 : Inport  Port=2
  rvalid_1 : Inport  Port=3
  rlast_1 : Inport  Port=4
  rdata_1 : Inport  Port=5
  rresp_1 : Inport  Port=6
  arready_2 : Inport  Port=7
  rvalid_2 : Inport  Port=8
  rlast_2 : Inport  Port=9
  rdata_2 : Inport  Port=10
  rresp_2 : Inport  Port=11
  Mux{,1..4} (5 alike) : xbsIndex_r4/Mux  inputs=2  en=off  latency=0  precision=Full  arith_type=Unsigned  n_bits=16  bin_pt=14  quantization=Truncate  overflow=Wrap  dbl_ovrd=off  block_type=mux
      settings: block_version=12.3
  arready : Outport
  rvalid : Outport  Port=2
  rlast : Outport  Port=3
  rdata : Outport  Port=4
  rresp : Outport  Port=5
  wires:
  gate/1 -> Mux/1, Mux1/1, Mux2/1, Mux3/1, Mux4/1
  arready_1/1 -> Mux/2
  Mux/1 -> arready/1
  arready_2/1 -> Mux/3
  rvalid_1/1 -> Mux1/2
  Mux1/1 -> rvalid/1
  rvalid_2/1 -> Mux1/3
  rlast_1/1 -> Mux2/2
  Mux2/1 -> rlast/1
  rlast_2/1 -> Mux2/3
  rdata_1/1 -> Mux3/2
  Mux3/1 -> rdata/1
  rdata_2/1 -> Mux3/3
  rresp_1/1 -> Mux4/2
  Mux4/1 -> rresp/1
  rresp_2/1 -> Mux4/3

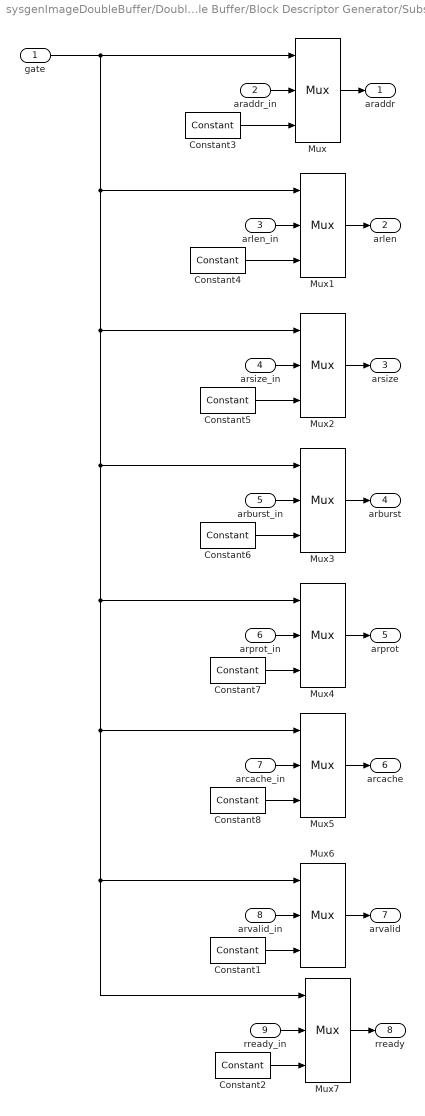
== system sysgenImageDoubleBuffer/Double Buffer/Double Buffer/Block Descriptor Generator/Subsystem4 ==
  gate : Inport
  araddr_in : Inport  Port=2
  arlen_in : Inport  Port=3
  arsize_in : Inport  Port=4
  arburst_in : Inport  Port=5
  arprot_in : Inport  Port=6
  arcache_in : Inport  Port=7
  arvalid_in : Inport  Port=8
  rready_in : Inport  Port=9
  Constant1 : xbsIndex_r4/Constant  const=0  gui_display_data_type=Fixed-point  arith_type=Boolean  n_bits=4  bin_pt=0  preci_type=Single  exp_width=8  frac_width=24  explicit_period=off  period=1  equ=P=C  opselect=C  inp2=PCIN>>17  opr=+  inp1=P  carry=CIN  dbl_ovrd=off  block_type=constant
      settings: block_version=12.3
  Constant2 : xbsIndex_r4/Constant  const=0  gui_display_data_type=Fixed-point  arith_type=Boolean  n_bits=4  bin_pt=0  preci_type=Single  exp_width=8  frac_width=24  explicit_period=off  period=1  equ=P=C  opselect=C  inp2=PCIN>>17  opr=+  inp1=P  carry=CIN  dbl_ovrd=off  block_type=constant
      settings: block_version=12.3
  Constant3 : xbsIndex_r4/Constant  const=0  gui_display_data_type=Fixed-point  arith_type=Unsigned  n_bits=32  bin_pt=0  preci_type=Single  exp_width=8  frac_width=24  explicit_period=off  period=1  equ=P=C  opselect=C  inp2=PCIN>>17  opr=+  inp1=P  carry=CIN  dbl_ovrd=off  block_type=constant
      settings: block_version=12.3
  Constant4 : xbsIndex_r4/Constant  const=0  gui_display_data_type=Fixed-point  arith_type=Unsigned  n_bits=8  bin_pt=0  preci_type=Single  exp_width=8  frac_width=24  explicit_period=off  period=1  equ=P=C  opselect=C  inp2=PCIN>>17  opr=+  inp1=P  carry=CIN  dbl_ovrd=off  block_type=constant
      settings: block_version=12.3
  Constant5 : xbsIndex_r4/Constant  const=0  gui_display_data_type=Fixed-point  arith_type=Unsigned  n_bits=3  bin_pt=0  preci_type=Single  exp_width=8  frac_width=24  explicit_period=off  period=1  equ=P=C  opselect=C  inp2=PCIN>>17  opr=+  inp1=P  carry=CIN  dbl_ovrd=off  block_type=constant
      settings: block_version=12.3
  Constant6 : xbsIndex_r4/Constant  const=0  gui_display_data_type=Fixed-point  arith_type=Unsigned  n_bits=2  bin_pt=0  preci_type=Single  exp_width=8  frac_width=24  explicit_period=off  period=1  equ=P=C  opselect=C  inp2=PCIN>>17  opr=+  inp1=P  carry=CIN  dbl_ovrd=off  block_type=constant
      settings: block_version=12.3
  Constant7 : xbsIndex_r4/Constant  const=0  gui_display_data_type=Fixed-point  arith_type=Unsigned  n_bits=3  bin_pt=0  preci_type=Single  exp_width=8  frac_width=24  explicit_period=off  period=1  equ=P=C  opselect=C  inp2=PCIN>>17  opr=+  inp1=P  carry=CIN  dbl_ovrd=off  block_type=constant
      settings: block_version=12.3
  Constant8 : xbsIndex_r4/Constant  const=0  gui_display_data_type=Fixed-point  arith_type=Unsigned  n_bits=4  bin_pt=0  preci_type=Single  exp_width=8  frac_width=24  explicit_period=off  period=1  equ=P=C  opselect=C  inp2=PCIN>>17  opr=+  inp1=P  carry=CIN  dbl_ovrd=off  block_type=constant
      settings: block_version=12.3
  Mux{,1..7} (8 alike) : xbsIndex_r4/Mux  inputs=2  en=off  latency=0  precision=Full  arith_type=Unsigned  n_bits=16  bin_pt=14  quantization=Truncate  overflow=Wrap  dbl_ovrd=off  block_type=mux
      settings: block_version=12.3
  araddr : Outport
  arlen : Outport  Port=2
  arsize : Outport  Port=3
  arburst : Outport  Port=4
  arprot : Outport  Port=5
  arcache : Outport  Port=6
  arvalid : Outport  Port=7
  rready : Outport  Port=8
  wires:
  Mux7/1 -> rready/1
  rready_in/1 -> Mux7/2
  Constant2/1 -> Mux7/3
  Mux6/1 -> arvalid/1
  arvalid_in/1 -> Mux6/2
  Constant1/1 -> Mux6/3
  Mux5/1 -> arcache/1
  arcache_in/1 -> Mux5/2
  Mux4/1 -> arprot/1
  arprot_in/1 -> Mux4/2
  Mux3/1 -> arburst/1
  arburst_in/1 -> Mux3/2
  Mux2/1 -> arsize/1
  arsize_in/1 -> Mux2/2
  Mux1/1 -> arlen/1
  arlen_in/1 -> Mux1/2
  Mux/1 -> araddr/1
  araddr_in/1 -> Mux/2
  gate/1 -> Mux7/1, Mux6/1, Mux5/1, Mux4/1, Mux3/1, Mux2/1, Mux1/1, Mux/1
  Constant8/1 -> Mux5/3
  Constant7/1 -> Mux4/3
  Constant6/1 -> Mux3/3
  Constant5/1 -> Mux2/3
  Constant4/1 -> Mux1/3
  Constant3/1 -> Mux/3
